simulink model "Appl_DrComfort_CtrlModel"  (R2018b)
settings: configuration reference "CodeConfig_10_ms" (kept outside this file)
undefined symbols (not defined in the file): D_Active, D_CLOSE, D_Inactive, D_InitDelayTime, D_OPEN, D_SoftDistanceDrLegnth, D_WelcomeDistance, FALSE, TRUE
libraries: DareLib x50, simulink x1
(part 1 of 2)
settings Model: Creator=Administrator  LastModifiedBy=Administrator
settings ConfigSetRef: SourceLocation=Base Workspace

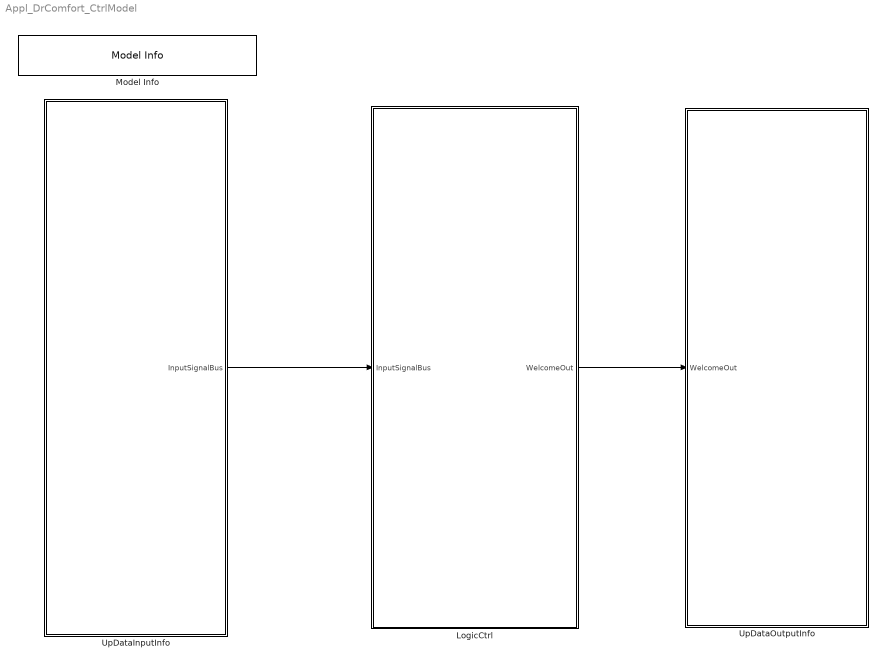
== system Appl_DrComfort_CtrlModel ==
  LogicCtrl : Subsystem  Priority=2  TreatAsAtomicUnit=on
      settings: RTWSystemCode=Nonreusable function  RTWFcnNameOpts=Use subsystem name
  Model Info : simulink/Model-Wide Utilities/Model Info  Frame=on  DisplayStringWithTags=Version：%<ModelVersion>  HorizontalTextAlignment=Center  LeftAlignmentValue=0.5
  UpDataInputInfo : Subsystem  Priority=1  TreatAsAtomicUnit=on
      settings: RTWSystemCode=Nonreusable function  RTWFcnNameOpts=Use subsystem name
  UpDataOutputInfo : Subsystem  Priority=3  TreatAsAtomicUnit=on
      settings: RTWSystemCode=Nonreusable function  RTWFcnNameOpts=Use subsystem name
  wires:
  LogicCtrl/1(WelcomeOut) -> UpDataOutputInfo/1(WelcomeOut)
  UpDataInputInfo/1(InputSignalBus) -> LogicCtrl/1(InputSignalBus)

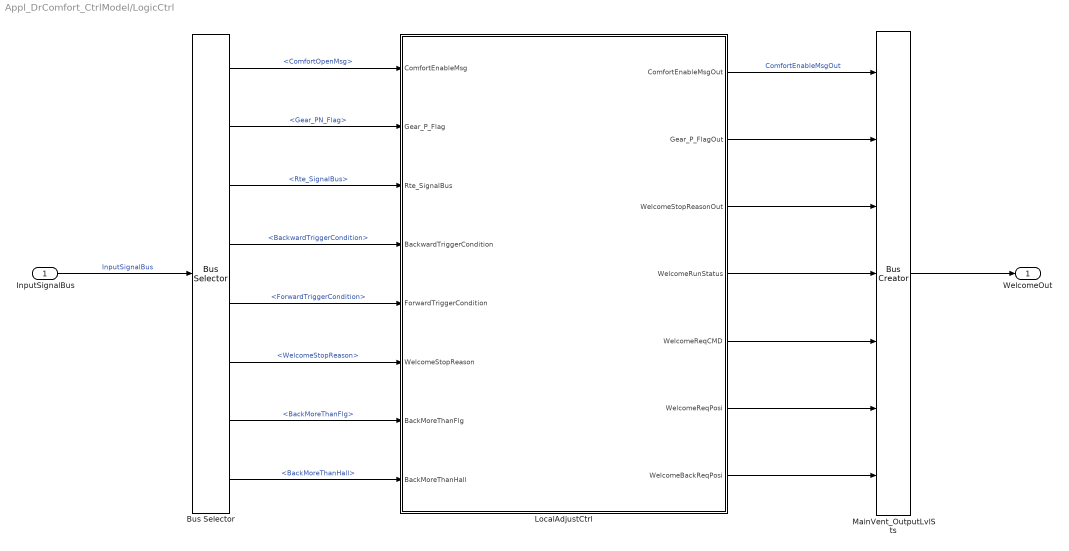
== system Appl_DrComfort_CtrlModel/LogicCtrl ==
  InputSignalBus : Inport
  Bus Selector : BusSelector  OutputSignals=ComfortOpenMsg,Gear_PN_Flag,Rte_SignalBus,BackwardTriggerCondition,ForwardTriggerCondition,WelcomeStopReason,BackMoreThanFlg,BackMoreThanHall
  LocalAdjustCtrl : Subsystem  Description=加热逻辑处理
      settings: AttributesFormatString=%<Description>
  MainVent_OutputLvlSts : BusCreator  Inputs=7
  WelcomeOut : Outport
  wires:
  InputSignalBus/1 -> Bus Selector/1  "InputSignalBus"
  MainVent_OutputLvlSts/1 -> WelcomeOut/1
  Bus Selector/3 -> LocalAdjustCtrl/3(Rte_SignalBus)  "<Rte_SignalBus>"
  Bus Selector/2 -> LocalAdjustCtrl/2(Gear_P_Flag)  "<Gear_PN_Flag>"
  Bus Selector/4 -> LocalAdjustCtrl/4(BackwardTriggerCondition)  "<BackwardTriggerCondition>"
  Bus Selector/5 -> LocalAdjustCtrl/5(ForwardTriggerCondition)  "<ForwardTriggerCondition>"
  Bus Selector/6 -> LocalAdjustCtrl/6(WelcomeStopReason)  "<WelcomeStopReason>"
  LocalAdjustCtrl/2(Gear_P_FlagOut) -> MainVent_OutputLvlSts/2
  LocalAdjustCtrl/3(WelcomeStopReasonOut) -> MainVent_OutputLvlSts/3
  LocalAdjustCtrl/4(WelcomeRunStatus) -> MainVent_OutputLvlSts/4
  LocalAdjustCtrl/5(WelcomeReqCMD) -> MainVent_OutputLvlSts/5
  LocalAdjustCtrl/6(WelcomeReqPosi) -> MainVent_OutputLvlSts/6
  Bus Selector/1 -> LocalAdjustCtrl/1(ComfortEnableMsg)  "<ComfortOpenMsg>"
  LocalAdjustCtrl/1(ComfortEnableMsgOut) -> MainVent_OutputLvlSts/1  "ComfortEnableMsgOut"
  Bus Selector/7 -> LocalAdjustCtrl/7(BackMoreThanFlg)  "<BackMoreThanFlg>"
  Bus Selector/8 -> LocalAdjustCtrl/8(BackMoreThanHall)  "<BackMoreThanHall>"
  LocalAdjustCtrl/7(WelcomeBackReqPosi) -> MainVent_OutputLvlSts/7

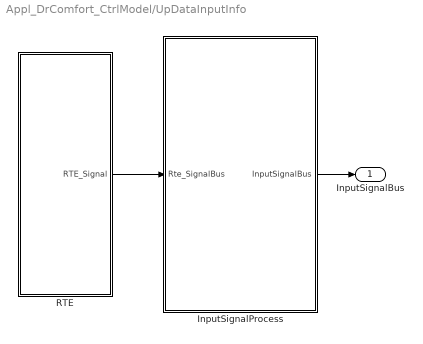
== system Appl_DrComfort_CtrlModel/UpDataInputInfo ==
  InputSignalProcess : Subsystem  Description=数据处理
      settings: AttributesFormatString=%<Description>  RTWSystemCode=Nonreusable function  RTWFcnNameOpts=Use subsystem name
  RTE : Subsystem  Description=接口自动生成  TreatAsAtomicUnit=on
      settings: AttributesFormatString=%<Description>  RTWSystemCode=Nonreusable function  RTWFcnNameOpts=Use subsystem name
  InputSignalBus : Outport
  wires:
  RTE/1(RTE_Signal) -> InputSignalProcess/1(Rte_SignalBus)
  InputSignalProcess/1(InputSignalBus) -> InputSignalBus/1

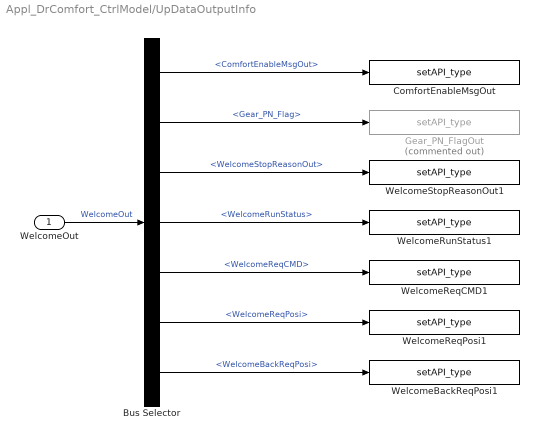
== system Appl_DrComfort_CtrlModel/UpDataOutputInfo ==
  WelcomeOut : Inport
  Bus Selector : BusSelector  OutputSignals=ComfortEnableMsgOut,Gear_PN_Flag,WelcomeStopReasonOut,WelcomeRunStatus,WelcomeReqCMD,WelcomeReqPosi,WelcomeBackReqPosi
  ComfortEnableMsgOut : DareLib/Dare/setAPI_type  g_funcname=CanTx_0x3B2_DSM_St_FLSeatmeet  g_param=""  g_type=uint8  g_size=-1
      settings: AttributesFormatString=%<g_funcname>  SourceProductName=Dare Library
  Gear_PN_FlagOut : DareLib/Dare/setAPI_type  Commented=on  g_funcname=Srvl_Set_D_SimuIndex_GearPN  g_param=D_SimuIndex_GearPN  g_type=uint8  g_size=-1
      settings: AttributesFormatString=%<g_funcname>  SourceProductName=Dare Library
  WelcomeBackReqPosi1 : DareLib/Dare/setAPI_type  g_funcname=Rte_SetVfb_DrWelBackReqPosi  g_param=""  g_type=uint16  g_size=-1
      settings: AttributesFormatString=%<g_funcname>  SourceProductName=Dare Library
  WelcomeReqCMD1 : DareLib/Dare/setAPI_type  g_funcname=Rte_SetVfb_DrWelLengthReqCMD  g_param=""  g_type=uint8  g_size=-1
      settings: AttributesFormatString=%<g_funcname>  SourceProductName=Dare Library
  WelcomeReqPosi1 : DareLib/Dare/setAPI_type  g_funcname=Rte_SetVfb_DrWelLengthReqPosi  g_param=""  g_type=uint16  g_size=-1
      settings: AttributesFormatString=%<g_funcname>  SourceProductName=Dare Library
  WelcomeRunStatus1 : DareLib/Dare/setAPI_type  g_funcname=Rte_SetVfb_DrWelcomeRunSts  g_param=""  g_type=uint8  g_size=-1
      settings: AttributesFormatString=%<g_funcname>  SourceProductName=Dare Library
  WelcomeStopReasonOut1 : DareLib/Dare/setAPI_type  g_funcname=Rte_SetVfb_DrWelcomeStopReason  g_param=""  g_type=uint8  g_size=-1
      settings: AttributesFormatString=%<g_funcname>  SourceProductName=Dare Library
  wires:
  WelcomeOut/1 -> Bus Selector/1  "WelcomeOut"
  Bus Selector/5 -> WelcomeReqCMD1/1  "<WelcomeReqCMD>"
  Bus Selector/4 -> WelcomeRunStatus1/1  "<WelcomeRunStatus>"
  Bus Selector/3 -> WelcomeStopReasonOut1/1  "<WelcomeStopReasonOut>"
  Bus Selector/2 -> Gear_PN_FlagOut/1  "<Gear_PN_Flag>"
  Bus Selector/6 -> WelcomeReqPosi1/1  "<WelcomeReqPosi>"
  Bus Selector/1 -> ComfortEnableMsgOut/1  "<ComfortEnableMsgOut>"
  Bus Selector/7 -> WelcomeBackReqPosi1/1  "<WelcomeBackReqPosi>"

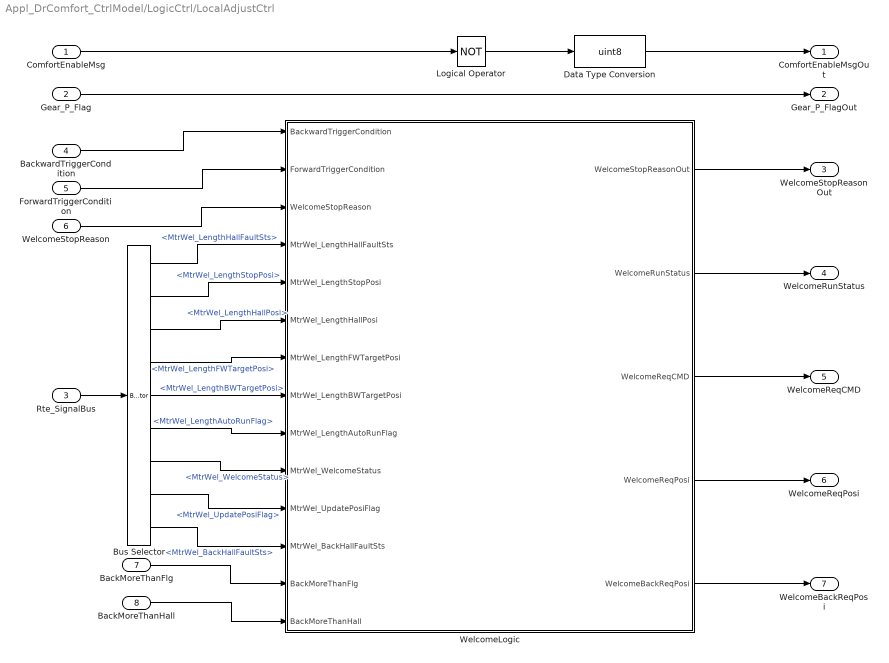
== system Appl_DrComfort_CtrlModel/LogicCtrl/LocalAdjustCtrl ==
  ComfortEnableMsg : Inport
  Gear_P_Flag : Inport  Port=2
  Rte_SignalBus : Inport  Port=3
  BackwardTriggerCondition : Inport  Port=4
  ForwardTriggerCondition : Inport  Port=5
  WelcomeStopReason : Inport  Port=6
  BackMoreThanFlg : Inport  Port=7
  BackMoreThanHall : Inport  Port=8
  Bus Selector : BusSelector  OutputSignals=MtrWel_LengthHallFaultSts,MtrWel_LengthStopPosi,MtrWel_LengthHallPosi,MtrWel_LengthFWTargetPosi,MtrWel_LengthBWTargetPosi,MtrWel_LengthAutoRunFlag,MtrWel_WelcomeStatus,MtrWel_UpdatePosiFlag,MtrWel_BackHallFaultSts
  Data Type Conversion : DataTypeConversion  OutDataTypeStr=uint8
  Logical Operator : Logic  Operator=NOT  AllPortsSameDT=off  OutDataTypeStr=boolean
  WelcomeLogic : Stateflow chart  TreatAsAtomicUnit=on
  ComfortEnableMsgOut : Outport
  Gear_P_FlagOut : Outport  Port=2
  WelcomeStopReasonOut : Outport  Port=3
  WelcomeRunStatus : Outport  Port=4
  WelcomeReqCMD : Outport  Port=5
  WelcomeReqPosi : Outport  Port=6
  WelcomeBackReqPosi : Outport  Port=7
  wires:
  Gear_P_Flag/1 -> Gear_P_FlagOut/1
  Rte_SignalBus/1 -> Bus Selector/1
  BackwardTriggerCondition/1 -> WelcomeLogic/1(BackwardTriggerCondition)
  ForwardTriggerCondition/1 -> WelcomeLogic/2(ForwardTriggerCondition)
  WelcomeStopReason/1 -> WelcomeLogic/3(WelcomeStopReason)
  Bus Selector/2 -> WelcomeLogic/5(MtrWel_LengthStopPosi)  "<MtrWel_LengthStopPosi>"
  Bus Selector/3 -> WelcomeLogic/6(MtrWel_LengthHallPosi)  "<MtrWel_LengthHallPosi>"
  Bus Selector/6 -> WelcomeLogic/9(MtrWel_LengthAutoRunFlag)  "<MtrWel_LengthAutoRunFlag>"
  Bus Selector/4 -> WelcomeLogic/7(MtrWel_LengthFWTargetPosi)  "<MtrWel_LengthFWTargetPosi>"
  Bus Selector/5 -> WelcomeLogic/8(MtrWel_LengthBWTargetPosi)  "<MtrWel_LengthBWTargetPosi>"
  Bus Selector/7 -> WelcomeLogic/10(MtrWel_WelcomeStatus)  "<MtrWel_WelcomeStatus>"
  WelcomeLogic/1(WelcomeStopReasonOut) -> WelcomeStopReasonOut/1
  WelcomeLogic/2(WelcomeRunStatus) -> WelcomeRunStatus/1
  WelcomeLogic/3(WelcomeReqCMD) -> WelcomeReqCMD/1
  WelcomeLogic/4(WelcomeReqPosi) -> WelcomeReqPosi/1
  Logical Operator/1 -> Data Type Conversion/1
  ComfortEnableMsg/1 -> Logical Operator/1
  Data Type Conversion/1 -> ComfortEnableMsgOut/1
  Bus Selector/1 -> WelcomeLogic/4(MtrWel_LengthHallFaultSts)  "<MtrWel_LengthHallFaultSts>"
  Bus Selector/8 -> WelcomeLogic/11(MtrWel_UpdatePosiFlag)  "<MtrWel_UpdatePosiFlag>"
  BackMoreThanHall/1 -> WelcomeLogic/14(BackMoreThanHall)
  BackMoreThanFlg/1 -> WelcomeLogic/13(BackMoreThanFlg)
  Bus Selector/9 -> WelcomeLogic/12(MtrWel_BackHallFaultSts)  "<MtrWel_BackHallFaultSts>"
  WelcomeLogic/5(WelcomeBackReqPosi) -> WelcomeBackReqPosi/1

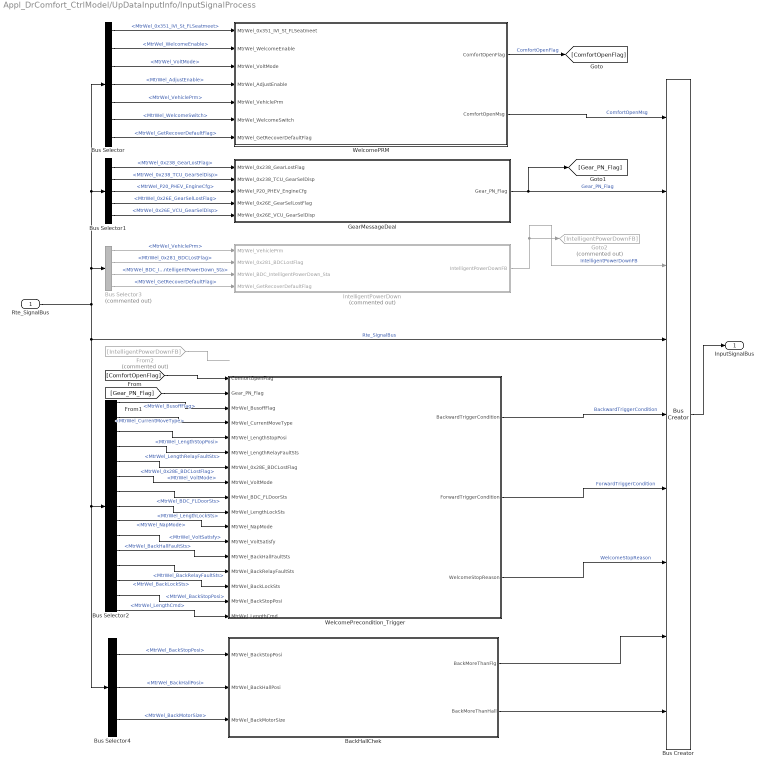
== system Appl_DrComfort_CtrlModel/UpDataInputInfo/InputSignalProcess ==
  Rte_SignalBus : Inport
  "BackHallChek " : Subsystem
  Bus Creator : BusCreator  Inputs=9
  Bus Selector : BusSelector  OutputSignals=MtrWel_0x351_IVI_St_FLSeatmeet,MtrWel_WelcomeEnable,MtrWel_VoltMode,MtrWel_AdjustEnable,MtrWel_VehiclePrm,MtrWel_WelcomeSwitch,MtrWel_GetRecoverDefaultFlag
  Bus Selector1 : BusSelector  OutputSignals=MtrWel_0x238_GearLostFlag,MtrWel_0x238_TCU_GearSelDisp,MtrWel_P20_PHEV_EngineCfg,MtrWel_0x26E_GearSelLostFlag,MtrWel_0x26E_VCU_GearSelDisp
  Bus Selector2 : BusSelector  OutputSignals=MtrWel_BusoffFlag,MtrWel_CurrentMoveType,MtrWel_LengthStopPosi,MtrWel_LengthRelayFaultSts,MtrWel_0x28E_BDCLostFlag,MtrWel_VoltMode,MtrWel_BDC_FLDoorSts,MtrWel_LengthLockSts,MtrWel_NapMode,MtrWel_VoltSatisfy,MtrWel_BackHallFaultSts,MtrWel_BackRelayFaultSts,MtrWel_BackLockSts,MtrWel_BackStopPosi,MtrWel_LengthCmd
  Bus Selector3 : BusSelector  Commented=on  OutputSignals=MtrWel_VehiclePrm,MtrWel_0x281_BDCLostFlag,MtrWel_BDC_IntelligentPowerDown_Sta,MtrWel_GetRecoverDefaultFlag
  Bus Selector4 : BusSelector  OutputSignals=MtrWel_BackStopPosi,MtrWel_BackHallPosi,MtrWel_BackMotorSize
  From2 : From  Commented=on  GotoTag=IntelligentPowerDownFB
  GearMessageDeal : Subsystem  Description=档位报文处理
      settings: AttributesFormatString=%<Description>
  Goto2 : Goto  Commented=on  GotoTag=IntelligentPowerDownFB
  IntelligentPowerDown : Subsystem  Description=智能下电处理  Commented=on
      settings: AttributesFormatString=%<Description>
  WelcomePRM : Subsystem  Description=迎宾配置
      settings: AttributesFormatString=%<Description>
  WelcomePrecondition_Trigger : Subsystem  Description=迎宾前置条件_触发条件
      settings: AttributesFormatString=%<Description>
  InputSignalBus : Outport
  wires:
  Bus Creator/1 -> InputSignalBus/1
  Rte_SignalBus/1 -> Bus Selector4/1, Bus Selector2/1, Bus Creator/4, Bus Selector/1, Bus Selector1/1, Bus Selector3/1  "Rte_SignalBus"
  WelcomePRM/1(ComfortOpenFlag) -> [ComfortOpenFlag]  "ComfortOpenFlag"
  Bus Selector/1 -> WelcomePRM/1(MtrWel_0x351_IVI_St_FLSeatmeet)  "<MtrWel_0x351_IVI_St_FLSeatmeet>"
  Bus Selector/2 -> WelcomePRM/2(MtrWel_WelcomeEnable)  "<MtrWel_WelcomeEnable>"
  Bus Selector/3 -> WelcomePRM/3(MtrWel_VoltMode)  "<MtrWel_VoltMode>"
  Bus Selector1/1 -> GearMessageDeal/1(MtrWel_0x238_GearLostFlag)  "<MtrWel_0x238_GearLostFlag>"
  Bus Selector1/2 -> GearMessageDeal/2(MtrWel_0x238_TCU_GearSelDisp)  "<MtrWel_0x238_TCU_GearSelDisp>"
  GearMessageDeal/1(Gear_PN_Flag) -> [Gear_PN_Flag], Bus Creator/2  "Gear_PN_Flag"
  Bus Selector2/1 -> WelcomePrecondition_Trigger/3(MtrWel_BusoffFlag)  "<MtrWel_BusoffFlag>"
  [Gear_PN_Flag] -> WelcomePrecondition_Trigger/2(Gear_PN_Flag)
  [ComfortOpenFlag] -> WelcomePrecondition_Trigger/1(ComfortOpenFlag)
  WelcomePrecondition_Trigger/1(BackwardTriggerCondition) -> Bus Creator/5  "BackwardTriggerCondition"
  WelcomePrecondition_Trigger/2(ForwardTriggerCondition) -> Bus Creator/6  "ForwardTriggerCondition"
  WelcomePrecondition_Trigger/3(WelcomeStopReason) -> Bus Creator/7  "WelcomeStopReason"
  Bus Selector2/2 -> WelcomePrecondition_Trigger/4(MtrWel_CurrentMoveType)  "<MtrWel_CurrentMoveType>"
  Bus Selector/4 -> WelcomePRM/4(MtrWel_AdjustEnable)  "<MtrWel_AdjustEnable>"
  Bus Selector/5 -> WelcomePRM/5(MtrWel_VehiclePrm)  "<MtrWel_VehiclePrm>"
  Bus Selector/6 -> WelcomePRM/6(MtrWel_WelcomeSwitch)  "<MtrWel_WelcomeSwitch>"
  Bus Selector/7 -> WelcomePRM/7(MtrWel_GetRecoverDefaultFlag)  "<MtrWel_GetRecoverDefaultFlag>"
  Bus Selector3/2 -> IntelligentPowerDown/2(MtrWel_0x281_BDCLostFlag)  "<MtrWel_0x281_BDCLostFlag>"
  Bus Selector3/3 -> IntelligentPowerDown/3(MtrWel_BDC_IntelligentPowerDown_Sta)  "<MtrWel_BDC_IntelligentPowerDown_Sta>"
  Bus Selector3/1 -> IntelligentPowerDown/1(MtrWel_VehiclePrm)  "<MtrWel_VehiclePrm>"
  IntelligentPowerDown/1(IntelligentPowerDownFB) -> Goto2/1, Bus Creator/3  "IntelligentPowerDownFB"
  From2/1 -> ?
  Bus Selector2/3 -> WelcomePrecondition_Trigger/5(MtrWel_LengthStopPosi)  "<MtrWel_LengthStopPosi>"
  Bus Selector2/4 -> WelcomePrecondition_Trigger/6(MtrWel_LengthRelayFaultSts)  "<MtrWel_LengthRelayFaultSts>"
  Bus Selector3/4 -> IntelligentPowerDown/4(MtrWel_GetRecoverDefaultFlag)  "<MtrWel_GetRecoverDefaultFlag>"
  Bus Selector2/5 -> WelcomePrecondition_Trigger/7(MtrWel_0x28E_BDCLostFlag)  "<MtrWel_0x28E_BDCLostFlag>"
  Bus Selector2/6 -> WelcomePrecondition_Trigger/8(MtrWel_VoltMode)  "<MtrWel_VoltMode>"
  Bus Selector2/7 -> WelcomePrecondition_Trigger/9(MtrWel_BDC_FLDoorSts)  "<MtrWel_BDC_FLDoorSts>"
  WelcomePRM/2(ComfortOpenMsg) -> Bus Creator/1  "ComfortOpenMsg"
  Bus Selector2/8 -> WelcomePrecondition_Trigger/10(MtrWel_LengthLockSts)  "<MtrWel_LengthLockSts>"
  Bus Selector2/9 -> WelcomePrecondition_Trigger/11(MtrWel_NapMode)  "<MtrWel_NapMode>"
  Bus Selector1/3 -> GearMessageDeal/3(MtrWel_P20_PHEV_EngineCfg)  "<MtrWel_P20_PHEV_EngineCfg>"
  Bus Selector1/4 -> GearMessageDeal/4(MtrWel_0x26E_GearSelLostFlag)  "<MtrWel_0x26E_GearSelLostFlag>"
  Bus Selector1/5 -> GearMessageDeal/5(MtrWel_0x26E_VCU_GearSelDisp)  "<MtrWel_0x26E_VCU_GearSelDisp>"
  Bus Selector2/10 -> WelcomePrecondition_Trigger/12(MtrWel_VoltSatisfy)  "<MtrWel_VoltSatisfy>"
  Bus Selector2/11 -> WelcomePrecondition_Trigger/13(MtrWel_BackHallFaultSts)  "<MtrWel_BackHallFaultSts>"
  Bus Selector2/12 -> WelcomePrecondition_Trigger/14(MtrWel_BackRelayFaultSts)  "<MtrWel_BackRelayFaultSts>"
  Bus Selector2/13 -> WelcomePrecondition_Trigger/15(MtrWel_BackLockSts)  "<MtrWel_BackLockSts>"
  Bus Selector2/14 -> WelcomePrecondition_Trigger/16(MtrWel_BackStopPosi)  "<MtrWel_BackStopPosi>"
  "BackHallChek "/1(BackMoreThanFlg) -> Bus Creator/8
  "BackHallChek "/2(BackMoreThanHall) -> Bus Creator/9
  Bus Selector4/1 -> "BackHallChek "/1(MtrWel_BackStopPosi)  "<MtrWel_BackStopPosi>"
  Bus Selector4/2 -> "BackHallChek "/2(MtrWel_BackHallPosi)  "<MtrWel_BackHallPosi>"
  Bus Selector4/3 -> "BackHallChek "/3(MtrWel_BackMotorSize)  "<MtrWel_BackMotorSize>"
  Bus Selector2/15 -> WelcomePrecondition_Trigger/17(MtrWel_LengthCmd)  "<MtrWel_LengthCmd>"

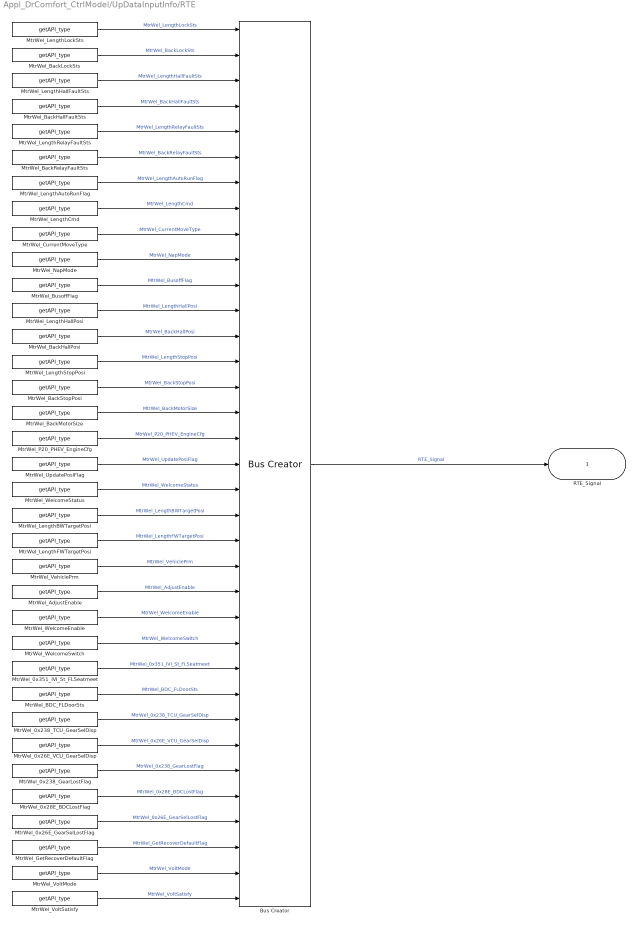
== system Appl_DrComfort_CtrlModel/UpDataInputInfo/RTE ==
  Bus Creator : BusCreator  Inputs=35
  MtrWel_0x238_GearLostFlag : DareLib/Dare/getAPI_type  g_funcname=Ecual_GetCanMsgLostFlag  g_param=eRXINDEX_0x238  g_type=uint8  g_size=-1
      settings: AttributesFormatString=%<g_funcname>  SourceProductName=Dare Library
  MtrWel_0x238_TCU_GearSelDisp : DareLib/Dare/getAPI_type  g_funcname=CanRx_0x238_TCU_GearSelDisp  g_param=""  g_type=uint8  g_size=-1
      settings: AttributesFormatString=%<g_funcname>  SourceProductName=Dare Library
  MtrWel_0x26E_GearSelLostFlag : DareLib/Dare/getAPI_type  g_funcname=Ecual_GetCanMsgLostFlag  g_param=eRXINDEX_0x26E  g_type=uint8  g_size=-1
      settings: AttributesFormatString=%<g_funcname>  SourceProductName=Dare Library
  MtrWel_0x26E_VCU_GearSelDisp : DareLib/Dare/getAPI_type  g_funcname=CanRx_0x26E_VCU_GearSelDisp  g_param=""  g_type=uint8  g_size=-1
      settings: AttributesFormatString=%<g_funcname>  SourceProductName=Dare Library
  MtrWel_0x28E_BDCLostFlag : DareLib/Dare/getAPI_type  g_funcname=Ecual_GetCanMsgLostFlag  g_param=eRXINDEX_0x28E  g_type=uint8  g_size=-1
      settings: AttributesFormatString=%<g_funcname>  SourceProductName=Dare Library
  MtrWel_0x351_IVI_St_FLSeatmeet : DareLib/Dare/getAPI_type  g_funcname=CanRx_0x351_IVI_St_FLSeatmeet  g_param=""  g_type=uint8  g_size=-1
      settings: AttributesFormatString=%<g_funcname>  SourceProductName=Dare Library
  MtrWel_AdjustEnable : DareLib/Dare/getAPI_type  g_funcname=Srvl_GetMemIndexDataU8  g_param=EN_MemIndex_DrAdjustConfig  g_type=uint8  g_enum=enDrAdjustEnable  g_size=-1
      settings: AttributesFormatString=%<g_funcname>  SourceProductName=Dare Library
  MtrWel_BDC_FLDoorSts : DareLib/Dare/getAPI_type  g_funcname=CanRx_0x28E_BDC_FLDoorSts  g_param=""  g_type=uint8  g_size=-1
      settings: AttributesFormatString=%<g_funcname>  SourceProductName=Dare Library
  MtrWel_BackHallFaultSts : DareLib/Dare/getAPI_type  g_funcname=Rte_GetVfb_DrBackHallErr  g_param=""  g_type=uint8  g_size=-1
      settings: AttributesFormatString=%<g_funcname>  SourceProductName=Dare Library
  MtrWel_BackHallPosi : DareLib/Dare/getAPI_type  g_funcname=Cdd_GetCurrentHallCnt  g_param=EN_DriverBack  g_type=uint16  g_size=-1
      settings: AttributesFormatString=%<g_funcname>  SourceProductName=Dare Library
  MtrWel_BackLockSts : DareLib/Dare/getAPI_type  g_funcname=Rte_GetVfb_DrBackStallErr  g_param=""  g_type=uint8  g_size=-1
      settings: AttributesFormatString=%<g_funcname>  SourceProductName=Dare Library
  MtrWel_BackMotorSize : DareLib/Dare/getAPI_type  g_funcname=Cdd_GetMotorSize  g_param=EN_DriverBack  g_type=uint16  g_size=-1
      settings: AttributesFormatString=%<g_funcname>  SourceProductName=Dare Library
  MtrWel_BackRelayFaultSts : DareLib/Dare/getAPI_type  g_funcname=Rte_GetVfb_DrBackRelayAdheErr  g_param=""  g_type=uint8  g_size=-1
      settings: AttributesFormatString=%<g_funcname>  SourceProductName=Dare Library
  MtrWel_BackStopPosi : DareLib/Dare/getAPI_type  g_funcname=Cdd_GetMotorHardStop  g_param=EN_DriverBack  g_type=uint16  g_size=-1
      settings: AttributesFormatString=%<g_funcname>  SourceProductName=Dare Library
  MtrWel_BusoffFlag : DareLib/Dare/getAPI_type  g_funcname=Nm_IsBusOff  g_param=""  g_type=uint8  g_size=-1
      settings: AttributesFormatString=%<g_funcname>  SourceProductName=Dare Library
  MtrWel_CurrentMoveType : DareLib/Dare/getAPI_type  g_funcname=Rte_GetVfb_DrMoveType  g_param=""  g_type=uint8  g_enum=enSeatMotorRunType  g_size=-1
      settings: AttributesFormatString=%<g_funcname>  SourceProductName=Dare Library
  MtrWel_GetRecoverDefaultFlag : DareLib/Dare/getAPI_type  g_funcname=GetRecoverDefaultFlag  g_param=""  g_type=uint8  g_size=-1
      settings: AttributesFormatString=%<g_funcname>  SourceProductName=Dare Library
  MtrWel_LengthAutoRunFlag : DareLib/Dare/getAPI_type  g_funcname=Rte_GetVfb_DrLengthAutoRunFlag  g_param=""  g_type=uint8  g_enum=enSeatAutoRunSts  g_size=-1
      settings: AttributesFormatString=%<g_funcname>  SourceProductName=Dare Library
  MtrWel_LengthBWTargetPosi : DareLib/Dare/getAPI_type  g_funcname=Srvl_GetMemIndexDataU16  g_param=EN_MemIndex_DrWelcome_LenTar_BackWard  g_type=uint16  g_size=-1
      settings: AttributesFormatString=%<g_funcname>  SourceProductName=Dare Library
  MtrWel_LengthCmd : DareLib/Dare/getAPI_type  g_funcname=Rte_GetVfb_DrHeightMotorCmd  g_param=""  g_type=uint8  g_size=-1
      settings: AttributesFormatString=%<g_funcname>  SourceProductName=Dare Library
  MtrWel_LengthFWTargetPosi : DareLib/Dare/getAPI_type  g_funcname=Srvl_GetMemIndexDataU16  g_param=EN_MemIndex_DrWelcome_LenTar_ForWard  g_type=uint16  g_size=-1
      settings: AttributesFormatString=%<g_funcname>  SourceProductName=Dare Library
  MtrWel_LengthHallFaultSts : DareLib/Dare/getAPI_type  g_funcname=Rte_GetVfb_DrLengthHallErr  g_param=""  g_type=uint8  g_size=-1
      settings: AttributesFormatString=%<g_funcname>  SourceProductName=Dare Library
  MtrWel_LengthHallPosi : DareLib/Dare/getAPI_type  g_funcname=Cdd_GetCurrentHallCnt  g_param=EN_DriverLength  g_type=uint16  g_size=-1
      settings: AttributesFormatString=%<g_funcname>  SourceProductName=Dare Library
  MtrWel_LengthLockSts : DareLib/Dare/getAPI_type  g_funcname=Rte_GetVfb_DrLengthStallErr  g_param=""  g_type=uint8  g_size=-1
      settings: AttributesFormatString=%<g_funcname>  SourceProductName=Dare Library
  MtrWel_LengthRelayFaultSts : DareLib/Dare/getAPI_type  g_funcname=Rte_GetVfb_DrLengthRelayAdheErr  g_param=""  g_type=uint8  g_size=-1
      settings: AttributesFormatString=%<g_funcname>  SourceProductName=Dare Library
  MtrWel_LengthStopPosi : DareLib/Dare/getAPI_type  g_funcname=Cdd_GetMotorHardStop  g_param=EN_DriverLength  g_type=uint16  g_size=-1
      settings: AttributesFormatString=%<g_funcname>  SourceProductName=Dare Library
  MtrWel_NapMode : DareLib/Dare/getAPI_type  g_funcname=Rte_GetVfb_NapMode  g_param=""  g_type=uint8  g_enum=enNapMode  g_size=-1
      settings: AttributesFormatString=%<g_funcname>  SourceProductName=Dare Library
  MtrWel_P20_PHEV_EngineCfg : DareLib/Dare/getAPI_type  g_funcname=Srvl_GetMemIndexDataU8  g_param=EN_MemIndex_Heat_P20_PHEV_EngineCfg  g_type=uint8  g_size=-1
      settings: AttributesFormatString=%<g_funcname>  SourceProductName=Dare Library
  MtrWel_UpdatePosiFlag : DareLib/Dare/getAPI_type  g_funcname=Srvl_GetMemIndexDataU8  g_param=EN_MemIndex_WelcomeDrUpate  g_type=uint8  g_size=-1
      settings: AttributesFormatString=%<g_funcname>  SourceProductName=Dare Library
  MtrWel_VehiclePrm : DareLib/Dare/getAPI_type  g_funcname=Srvl_GetMemIndexDataU8  g_param=EN_MemIndex_Heat_CarType  g_type=uint8  g_enum=enVehTypePrm  g_size=-1
      settings: AttributesFormatString=%<g_funcname>  SourceProductName=Dare Library
  MtrWel_VoltMode : DareLib/Dare/getAPI_type  g_funcname=Rte_GetVfb_VoltMode  g_param=""  g_type=uint8  g_enum=enFinalPowerMode  g_size=-1
      settings: AttributesFormatString=%<g_funcname>  SourceProductName=Dare Library
  MtrWel_VoltSatisfy : DareLib/Dare/getAPI_type  g_funcname=Rte_GetVfb_VoltSatisfy  g_param=""  g_type=uint8  g_size=-1
      settings: AttributesFormatString=%<g_funcname>  SourceProductName=Dare Library
  MtrWel_WelcomeEnable : DareLib/Dare/getAPI_type  g_funcname=Srvl_GetMemIndexDataU8  g_param=EN_MemIndex_DrMemoryConfig  g_type=uint8  g_size=-1
      settings: AttributesFormatString=%<g_funcname>  SourceProductName=Dare Library
  MtrWel_WelcomeStatus : DareLib/Dare/getAPI_type  g_funcname=Srvl_GetMemIndexDataU8  g_param=EN_MemIndex_WelcomeStatus  g_type=uint8  g_enum=enWelcomeSts  g_size=-1
      settings: AttributesFormatString=%<g_funcname>  SourceProductName=Dare Library
  MtrWel_WelcomeSwitch : DareLib/Dare/getAPI_type  g_funcname=Srvl_GetMemIndexDataU8  g_param=EN_MemIndex_WelcomeSwitch  g_type=uint8  g_size=-1
      settings: AttributesFormatString=%<g_funcname>  SourceProductName=Dare Library
  RTE_Signal : Outport
  wires:
  Bus Creator/1 -> RTE_Signal/1  "RTE_Signal"
  MtrWel_LengthLockSts/1 -> Bus Creator/1  "MtrWel_LengthLockSts"
  MtrWel_BackLockSts/1 -> Bus Creator/2  "MtrWel_BackLockSts"
  MtrWel_LengthHallFaultSts/1 -> Bus Creator/3  "MtrWel_LengthHallFaultSts"
  MtrWel_BackHallFaultSts/1 -> Bus Creator/4  "MtrWel_BackHallFaultSts"
  MtrWel_LengthRelayFaultSts/1 -> Bus Creator/5  "MtrWel_LengthRelayFaultSts"
  MtrWel_BackRelayFaultSts/1 -> Bus Creator/6  "MtrWel_BackRelayFaultSts"
  MtrWel_LengthAutoRunFlag/1 -> Bus Creator/7  "MtrWel_LengthAutoRunFlag"
  MtrWel_LengthCmd/1 -> Bus Creator/8  "MtrWel_LengthCmd"
  MtrWel_CurrentMoveType/1 -> Bus Creator/9  "MtrWel_CurrentMoveType"
  MtrWel_NapMode/1 -> Bus Creator/10  "MtrWel_NapMode"
  MtrWel_BusoffFlag/1 -> Bus Creator/11  "MtrWel_BusoffFlag"
  MtrWel_LengthHallPosi/1 -> Bus Creator/12  "MtrWel_LengthHallPosi"
  MtrWel_BackHallPosi/1 -> Bus Creator/13  "MtrWel_BackHallPosi"
  MtrWel_LengthStopPosi/1 -> Bus Creator/14  "MtrWel_LengthStopPosi"
  MtrWel_BackStopPosi/1 -> Bus Creator/15  "MtrWel_BackStopPosi"
  MtrWel_BackMotorSize/1 -> Bus Creator/16  "MtrWel_BackMotorSize"
  MtrWel_P20_PHEV_EngineCfg/1 -> Bus Creator/17  "MtrWel_P20_PHEV_EngineCfg"
  MtrWel_UpdatePosiFlag/1 -> Bus Creator/18  "MtrWel_UpdatePosiFlag"
  MtrWel_WelcomeStatus/1 -> Bus Creator/19  "MtrWel_WelcomeStatus"
  MtrWel_LengthBWTargetPosi/1 -> Bus Creator/20  "MtrWel_LengthBWTargetPosi"
  MtrWel_LengthFWTargetPosi/1 -> Bus Creator/21  "MtrWel_LengthFWTargetPosi"
  MtrWel_VehiclePrm/1 -> Bus Creator/22  "MtrWel_VehiclePrm"
  MtrWel_AdjustEnable/1 -> Bus Creator/23  "MtrWel_AdjustEnable"
  MtrWel_WelcomeEnable/1 -> Bus Creator/24  "MtrWel_WelcomeEnable"
  MtrWel_WelcomeSwitch/1 -> Bus Creator/25  "MtrWel_WelcomeSwitch"
  MtrWel_0x351_IVI_St_FLSeatmeet/1 -> Bus Creator/26  "MtrWel_0x351_IVI_St_FLSeatmeet"
  MtrWel_BDC_FLDoorSts/1 -> Bus Creator/27  "MtrWel_BDC_FLDoorSts"
  MtrWel_0x238_TCU_GearSelDisp/1 -> Bus Creator/28  "MtrWel_0x238_TCU_GearSelDisp"
  MtrWel_0x26E_VCU_GearSelDisp/1 -> Bus Creator/29  "MtrWel_0x26E_VCU_GearSelDisp"
  MtrWel_0x238_GearLostFlag/1 -> Bus Creator/30  "MtrWel_0x238_GearLostFlag"
  MtrWel_0x28E_BDCLostFlag/1 -> Bus Creator/31  "MtrWel_0x28E_BDCLostFlag"
  MtrWel_0x26E_GearSelLostFlag/1 -> Bus Creator/32  "MtrWel_0x26E_GearSelLostFlag"
  MtrWel_GetRecoverDefaultFlag/1 -> Bus Creator/33  "MtrWel_GetRecoverDefaultFlag"
  MtrWel_VoltMode/1 -> Bus Creator/34  "MtrWel_VoltMode"
  MtrWel_VoltSatisfy/1 -> Bus Creator/35  "MtrWel_VoltSatisfy"

== system Appl_DrComfort_CtrlModel/LogicCtrl/LocalAdjustCtrl/WelcomeLogic/Set_WelcomeBWTargertPosi ==
  In1 : Inport
  f : TriggerPort  TriggerType=function-call  VariantControl=(inherit)
      settings: CopyFcn=Stateflow.SLINSF.SimulinkMan.removeBlockPreDeleteFcn  PreDeleteFcn=Stateflow.SLINSF.SimulinkMan.unsafePredeleteFcn
  setAPI_type : DareLib/Dare/setAPI_type  g_funcname=Srvl_SetMemIndexDataU16  g_param=EN_MemIndex_DrWelcome_LenTar_BackWard  g_type=uint16  g_size=-1
      settings: AttributesFormatString=%<g_funcname>  SourceProductName=Dare Library
  wires:
  In1/1 -> setAPI_type/1

== system Appl_DrComfort_CtrlModel/LogicCtrl/LocalAdjustCtrl/WelcomeLogic/Set_WelcomeFWTargertPosi ==
  In1 : Inport
  f : TriggerPort  TriggerType=function-call  VariantControl=(inherit)
      settings: CopyFcn=Stateflow.SLINSF.SimulinkMan.removeBlockPreDeleteFcn  PreDeleteFcn=Stateflow.SLINSF.SimulinkMan.unsafePredeleteFcn
  setAPI_type : DareLib/Dare/setAPI_type  g_funcname=Srvl_SetMemIndexDataU16  g_param=EN_MemIndex_DrWelcome_LenTar_ForWard  g_type=uint16  g_size=-1
      settings: AttributesFormatString=%<g_funcname>  SourceProductName=Dare Library
  wires:
  In1/1 -> setAPI_type/1

== system Appl_DrComfort_CtrlModel/LogicCtrl/LocalAdjustCtrl/WelcomeLogic/Set_WelcomeStatus ==
  In1 : Inport
  f : TriggerPort  TriggerType=function-call  VariantControl=(inherit)
      settings: CopyFcn=Stateflow.SLINSF.SimulinkMan.removeBlockPreDeleteFcn  PreDeleteFcn=Stateflow.SLINSF.SimulinkMan.unsafePredeleteFcn
  setAPI_type : DareLib/Dare/setAPI_type  g_funcname=Srvl_SetMemIndexDataU8  g_param=EN_MemIndex_WelcomeStatus  g_type=uint8  g_size=-1
      settings: AttributesFormatString=%<g_funcname>  SourceProductName=Dare Library
  wires:
  In1/1 -> setAPI_type/1

== system Appl_DrComfort_CtrlModel/LogicCtrl/LocalAdjustCtrl/WelcomeLogic/Set_WelcomeUpdatePosiFlag ==
  In1 : Inport
  f : TriggerPort  TriggerType=function-call  VariantControl=(inherit)
      settings: CopyFcn=Stateflow.SLINSF.SimulinkMan.removeBlockPreDeleteFcn  PreDeleteFcn=Stateflow.SLINSF.SimulinkMan.unsafePredeleteFcn
  setAPI_type : DareLib/Dare/setAPI_type  g_funcname=Srvl_SetMemIndexDataU8  g_param=EN_MemIndex_WelcomeDrUpate  g_type=uint16  g_size=-1
      settings: AttributesFormatString=%<g_funcname>  SourceProductName=Dare Library
  wires:
  In1/1 -> setAPI_type/1

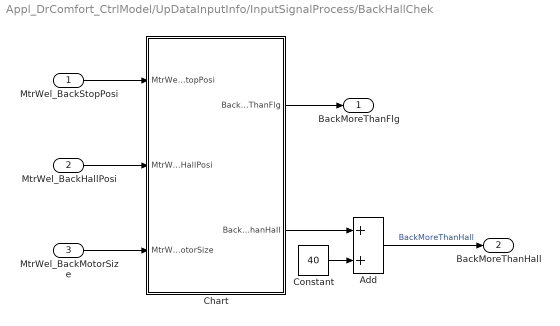
== system Appl_DrComfort_CtrlModel/UpDataInputInfo/InputSignalProcess/BackHallChek  ==
  MtrWel_BackStopPosi : Inport
  MtrWel_BackHallPosi : Inport  Port=2
  MtrWel_BackMotorSize : Inport  Port=3
  Add : Sum  AccumDataTypeStr=uint16
  Chart : Stateflow chart  TreatAsAtomicUnit=on
  Constant : Constant  Value=40  OutDataTypeStr=uint16
  BackMoreThanFlg : Outport
  BackMoreThanHall : Outport  Port=2
  wires:
  MtrWel_BackStopPosi/1 -> Chart/1(MtrWel_BackStopPosi)
  MtrWel_BackHallPosi/1 -> Chart/2(MtrWel_BackHallPosi)
  MtrWel_BackMotorSize/1 -> Chart/3(MtrWel_BackMotorSize)
  Chart/1(BackMoreThanFlg) -> BackMoreThanFlg/1
  Chart/2(BackMoreThanHall) -> Add/1
  Constant/1 -> Add/2
  Add/1 -> BackMoreThanHall/1  "BackMoreThanHall"

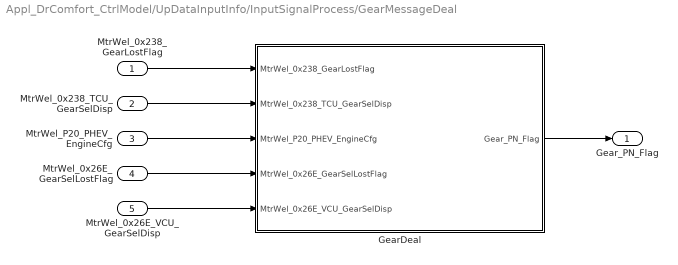
== system Appl_DrComfort_CtrlModel/UpDataInputInfo/InputSignalProcess/GearMessageDeal ==
  MtrWel_0x238_GearLostFlag : Inport
  MtrWel_0x238_TCU_GearSelDisp : Inport  Port=2
  MtrWel_P20_PHEV_EngineCfg : Inport  Port=3
  MtrWel_0x26E_GearSelLostFlag : Inport  Port=4
  MtrWel_0x26E_VCU_GearSelDisp : Inport  Port=5
  GearDeal : Stateflow chart  TreatAsAtomicUnit=on
  Gear_PN_Flag : Outport
  wires:
  MtrWel_0x238_GearLostFlag/1 -> GearDeal/1(MtrWel_0x238_GearLostFlag)
  MtrWel_0x238_TCU_GearSelDisp/1 -> GearDeal/2(MtrWel_0x238_TCU_GearSelDisp)
  GearDeal/1(Gear_PN_Flag) -> Gear_PN_Flag/1
  MtrWel_P20_PHEV_EngineCfg/1 -> GearDeal/3(MtrWel_P20_PHEV_EngineCfg)
  MtrWel_0x26E_GearSelLostFlag/1 -> GearDeal/4(MtrWel_0x26E_GearSelLostFlag)
  MtrWel_0x26E_VCU_GearSelDisp/1 -> GearDeal/5(MtrWel_0x26E_VCU_GearSelDisp)

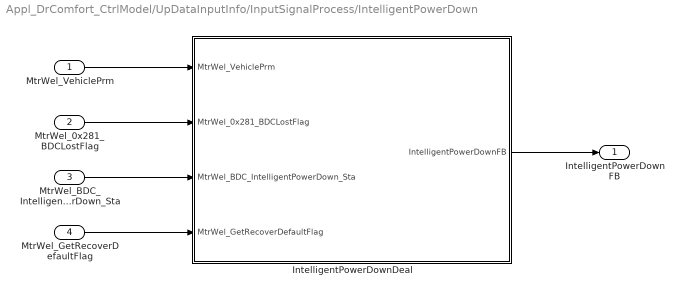
== system Appl_DrComfort_CtrlModel/UpDataInputInfo/InputSignalProcess/IntelligentPowerDown ==
  MtrWel_VehiclePrm : Inport
  MtrWel_0x281_BDCLostFlag : Inport  Port=2
  MtrWel_BDC_IntelligentPowerDown_Sta : Inport  Port=3
  MtrWel_GetRecoverDefaultFlag : Inport  Port=4
  IntelligentPowerDownDeal : Stateflow chart  TreatAsAtomicUnit=on
  IntelligentPowerDownFB : Outport
  wires:
  MtrWel_0x281_BDCLostFlag/1 -> IntelligentPowerDownDeal/2(MtrWel_0x281_BDCLostFlag)
  MtrWel_BDC_IntelligentPowerDown_Sta/1 -> IntelligentPowerDownDeal/3(MtrWel_BDC_IntelligentPowerDown_Sta)
  IntelligentPowerDownDeal/1(IntelligentPowerDownFB) -> IntelligentPowerDownFB/1
  MtrWel_VehiclePrm/1 -> IntelligentPowerDownDeal/1(MtrWel_VehiclePrm)
  MtrWel_GetRecoverDefaultFlag/1 -> IntelligentPowerDownDeal/4(MtrWel_GetRecoverDefaultFlag)

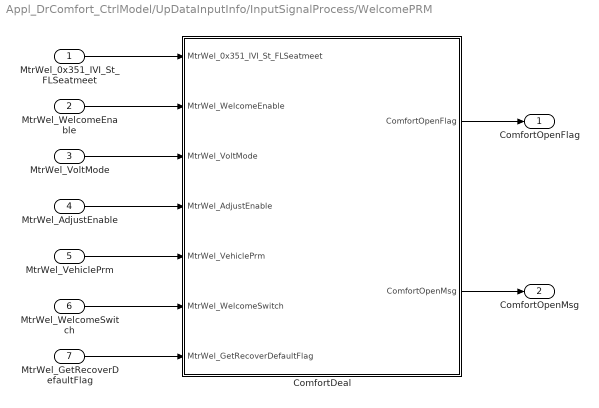
== system Appl_DrComfort_CtrlModel/UpDataInputInfo/InputSignalProcess/WelcomePRM ==
  MtrWel_0x351_IVI_St_FLSeatmeet : Inport
  MtrWel_WelcomeEnable : Inport  Port=2
  MtrWel_VoltMode : Inport  Port=3
  MtrWel_AdjustEnable : Inport  Port=4
  MtrWel_VehiclePrm : Inport  Port=5
  MtrWel_WelcomeSwitch : Inport  Port=6
  MtrWel_GetRecoverDefaultFlag : Inport  Port=7
  ComfortDeal : Stateflow chart  TreatAsAtomicUnit=on
  ComfortOpenFlag : Outport
  ComfortOpenMsg : Outport  Port=2
  wires:
  MtrWel_VoltMode/1 -> ComfortDeal/3(MtrWel_VoltMode)
  MtrWel_0x351_IVI_St_FLSeatmeet/1 -> ComfortDeal/1(MtrWel_0x351_IVI_St_FLSeatmeet)
  MtrWel_WelcomeEnable/1 -> ComfortDeal/2(MtrWel_WelcomeEnable)
  ComfortDeal/1(ComfortOpenFlag) -> ComfortOpenFlag/1
  MtrWel_AdjustEnable/1 -> ComfortDeal/4(MtrWel_AdjustEnable)
  MtrWel_VehiclePrm/1 -> ComfortDeal/5(MtrWel_VehiclePrm)
  MtrWel_WelcomeSwitch/1 -> ComfortDeal/6(MtrWel_WelcomeSwitch)
  MtrWel_GetRecoverDefaultFlag/1 -> ComfortDeal/7(MtrWel_GetRecoverDefaultFlag)
  ComfortDeal/2(ComfortOpenMsg) -> ComfortOpenMsg/1

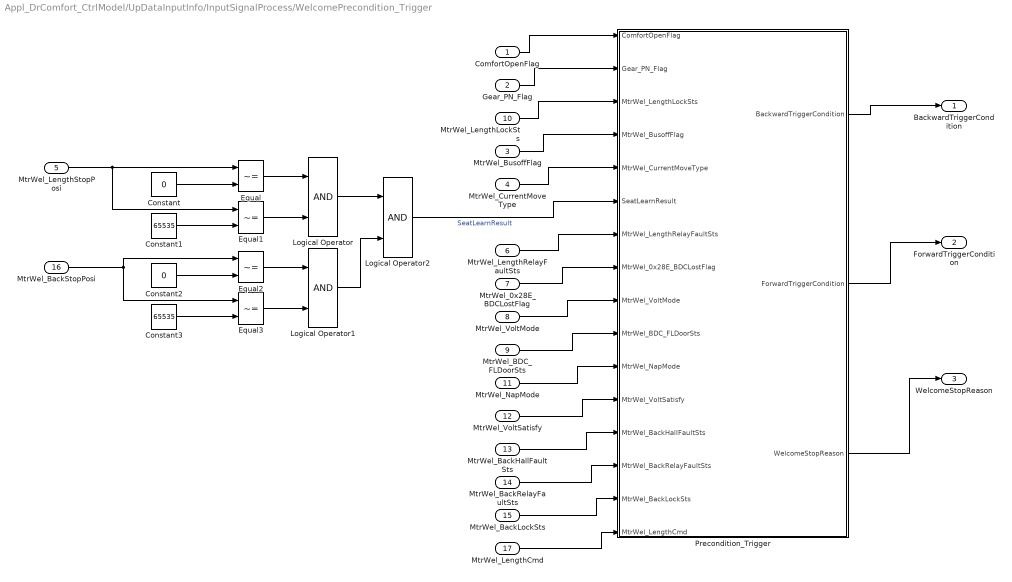
== system Appl_DrComfort_CtrlModel/UpDataInputInfo/InputSignalProcess/WelcomePrecondition_Trigger ==
  ComfortOpenFlag : Inport
  Gear_PN_Flag : Inport  Port=2
  MtrWel_BusoffFlag : Inport  Port=3
  MtrWel_CurrentMoveType : Inport  Port=4
  MtrWel_LengthStopPosi : Inport  Port=5
  MtrWel_LengthRelayFaultSts : Inport  Port=6
  MtrWel_0x28E_BDCLostFlag : Inport  Port=7
  MtrWel_VoltMode : Inport  Port=8
  MtrWel_BDC_FLDoorSts : Inport  Port=9
  MtrWel_LengthLockSts : Inport  Port=10
  MtrWel_NapMode : Inport  Port=11
  MtrWel_VoltSatisfy : Inport  Port=12
  MtrWel_BackHallFaultSts : Inport  Port=13
  MtrWel_BackRelayFaultSts : Inport  Port=14
  MtrWel_BackLockSts : Inport  Port=15
  MtrWel_BackStopPosi : Inport  Port=16
  MtrWel_LengthCmd : Inport  Port=17
  Constant : Constant  Value=0
  Constant1 : Constant  Value=65535
  Constant2 : Constant  Value=0
  Constant3 : Constant  Value=65535
  Equal{,1..3} (4 alike) : RelationalOperator  Operator=~=  OutDataTypeStr=boolean  RndMeth=Simplest
  Logical Operator : Logic  AllPortsSameDT=off  OutDataTypeStr=boolean
  Logical Operator1 : Logic  AllPortsSameDT=off  OutDataTypeStr=boolean
  Logical Operator2 : Logic  AllPortsSameDT=off  OutDataTypeStr=boolean
  Precondition_Trigger : Stateflow chart  TreatAsAtomicUnit=on
  BackwardTriggerCondition : Outport
  ForwardTriggerCondition : Outport  Port=2
  WelcomeStopReason : Outport  Port=3
  wires:
  MtrWel_BusoffFlag/1 -> Precondition_Trigger/4(MtrWel_BusoffFlag)
  Precondition_Trigger/1(BackwardTriggerCondition) -> BackwardTriggerCondition/1
  ComfortOpenFlag/1 -> Precondition_Trigger/1(ComfortOpenFlag)
  Gear_PN_Flag/1 -> Precondition_Trigger/2(Gear_PN_Flag)
  Precondition_Trigger/2(ForwardTriggerCondition) -> ForwardTriggerCondition/1
  Precondition_Trigger/3(WelcomeStopReason) -> WelcomeStopReason/1
  MtrWel_CurrentMoveType/1 -> Precondition_Trigger/5(MtrWel_CurrentMoveType)
  MtrWel_LengthRelayFaultSts/1 -> Precondition_Trigger/7(MtrWel_LengthRelayFaultSts)
  MtrWel_0x28E_BDCLostFlag/1 -> Precondition_Trigger/8(MtrWel_0x28E_BDCLostFlag)
  MtrWel_VoltMode/1 -> Precondition_Trigger/9(MtrWel_VoltMode)
  MtrWel_BDC_FLDoorSts/1 -> Precondition_Trigger/10(MtrWel_BDC_FLDoorSts)
  MtrWel_LengthLockSts/1 -> Precondition_Trigger/3(MtrWel_LengthLockSts)
  Constant1/1 -> Equal1/2
  Constant/1 -> Equal/2
  MtrWel_LengthStopPosi/1 -> Equal1/1, Equal/1
  Equal/1 -> Logical Operator/1
  Equal1/1 -> Logical Operator/2
  Logical Operator2/1 -> Precondition_Trigger/6(SeatLearnResult)  "SeatLearnResult"
  MtrWel_NapMode/1 -> Precondition_Trigger/11(MtrWel_NapMode)
  MtrWel_VoltSatisfy/1 -> Precondition_Trigger/12(MtrWel_VoltSatisfy)
  MtrWel_BackHallFaultSts/1 -> Precondition_Trigger/13(MtrWel_BackHallFaultSts)
  MtrWel_BackRelayFaultSts/1 -> Precondition_Trigger/14(MtrWel_BackRelayFaultSts)
  MtrWel_BackLockSts/1 -> Precondition_Trigger/15(MtrWel_BackLockSts)
  Logical Operator1/1 -> Logical Operator2/2
  Equal3/1 -> Logical Operator1/2
  Equal2/1 -> Logical Operator1/1
  MtrWel_BackStopPosi/1 -> Equal3/1, Equal2/1
  Constant2/1 -> Equal2/2
  Constant3/1 -> Equal3/2
  Logical Operator/1 -> Logical Operator2/1
  MtrWel_LengthCmd/1 -> Precondition_Trigger/16(MtrWel_LengthCmd)

== system Appl_DrComfort_CtrlModel/UpDataInputInfo/InputSignalProcess/WelcomePRM/ComfortDeal/SetComfortPrm ==
  in : Inport
  f : TriggerPort  TriggerType=function-call  VariantControl=(inherit)
      settings: CopyFcn=Stateflow.SLINSF.SimulinkMan.removeBlockPreDeleteFcn  PreDeleteFcn=Stateflow.SLINSF.SimulinkMan.unsafePredeleteFcn
  setAPI_type : DareLib/Dare/setAPI_type  g_funcname=Srvl_SetMemIndexDataU8  g_param=EN_MemIndex_WelcomeSwitch  g_type=uint8  g_size=-1
      settings: AttributesFormatString=%<g_funcname>  SourceProductName=Dare Library
  wires:
  in/1 -> setAPI_type/1

== system Appl_DrComfort_CtrlModel/UpDataInputInfo/InputSignalProcess/WelcomePrecondition_Trigger/Precondition_Trigger/Get_DoorSts ==
  f : TriggerPort  TriggerType=function-call  VariantControl=(inherit)
      settings: CopyFcn=Stateflow.SLINSF.SimulinkMan.removeBlockPreDeleteFcn  PreDeleteFcn=Stateflow.SLINSF.SimulinkMan.unsafePredeleteFcn
  MtrWel_WelcomeSwitch : DareLib/Dare/getAPI_type  g_funcname=Srvl_GetMemIndexDataU8  g_param=EN_MemIndex_DrDoorSts  g_type=uint8  g_size=-1
      settings: AttributesFormatString=%<g_funcname>  SourceProductName=Dare Library
  Out1 : Outport
  wires:
  MtrWel_WelcomeSwitch/1 -> Out1/1

== system Appl_DrComfort_CtrlModel/UpDataInputInfo/InputSignalProcess/WelcomePrecondition_Trigger/Precondition_Trigger/Set_DoorSts ==
  In1 : Inport
  f : TriggerPort  TriggerType=function-call  VariantControl=(inherit)
      settings: CopyFcn=Stateflow.SLINSF.SimulinkMan.removeBlockPreDeleteFcn  PreDeleteFcn=Stateflow.SLINSF.SimulinkMan.unsafePredeleteFcn
  setAPI_type : DareLib/Dare/setAPI_type  g_funcname=Srvl_SetMemIndexDataU8  g_param=EN_MemIndex_DrDoorSts  g_type=uint16  g_size=-1
      settings: AttributesFormatString=%<g_funcname>  SourceProductName=Dare Library
  wires:
  In1/1 -> setAPI_type/1

== system Appl_DrComfort_CtrlModel/UpDataInputInfo/InputSignalProcess/WelcomePrecondition_Trigger/Precondition_Trigger/Set_WelcomeUpdatePosiFlag ==
  In1 : Inport
  f : TriggerPort  TriggerType=function-call  VariantControl=(inherit)
      settings: CopyFcn=Stateflow.SLINSF.SimulinkMan.removeBlockPreDeleteFcn  PreDeleteFcn=Stateflow.SLINSF.SimulinkMan.unsafePredeleteFcn
  setAPI_type : DareLib/Dare/setAPI_type  g_funcname=Srvl_SetMemIndexDataU8  g_param=EN_MemIndex_WelcomeDrUpate  g_type=uint16  g_size=-1
      settings: AttributesFormatString=%<g_funcname>  SourceProductName=Dare Library
  wires:
  In1/1 -> setAPI_type/1

== stateflow chart Appl_DrComfort_CtrlModel/UpDataInputInfo/InputSignalProcess/IntelligentPowerDown/IntelligentPowerDownDeal ==
  state IntelligentPD_Active
    en:
    IntelligentPowerDownFB = D_Active;
  state IntelligentPD_Inactive
    en:
    IntelligentPowerDownFB = D_Inactive;
  note: /*BDC智能下电功能设置
      | 0x0:inactive
      | 0x1:active*/
  (default) -> IntelligentPD_Inactive
  IntelligentPD_Inactive -> IntelligentPD_Active : /*激活-打开*/
      | [D_Active == MtrWel_BDC_IntelligentPowerDown_Sta ...
      | && enVehTypePrm.enP20 == MtrWel_VehiclePrm]
  IntelligentPD_Active -> IntelligentPD_Inactive [order 1] : /*报文掉线 || 非激活-关闭 || 非P20车型*/
      | [TRUE == MtrWel_0x281_BDCLostFlag ...
      | || D_Inactive == MtrWel_BDC_IntelligentPowerDown_Sta ...
      | || enVehTypePrm.enP20 != MtrWel_VehiclePrm]
  IntelligentPD_Active -> IntelligentPD_Inactive [order 2] : [TRUE == MtrWel_GetRecoverDefaultFlag]
  data: MtrWel_VehiclePrm input; MtrWel_0x281_BDCLostFlag input; MtrWel_BDC_IntelligentPowerDown_Sta input; IntelligentPowerDownFB output uint8; TRUE parameter; D_Active parameter; D_Inactive parameter; MtrWel_GetRecoverDefaultFlag input

== stateflow chart Appl_DrComfort_CtrlModel/UpDataInputInfo/InputSignalProcess/BackHallChek /Chart ==
  state Check [parallel]
    en:
    BackMoreThanHall = MtrWel_BackStopPosi + (MtrWel_BackMotorSize / 4);
    du:
    BackMoreThanHall = MtrWel_BackStopPosi + (MtrWel_BackMotorSize / 4);
    settings: executionOrder=1
  state More [parallel]
    settings: executionOrder=2
    state Init
      en:
      BackMoreThanFlg = FALSE;
    state MoreThan
      en:
      BackMoreThanFlg = TRUE;
    (default) -> Init
    Init -> MoreThan : /* 大于距前止点60°位置 */
        | [MtrWel_BackHallPosi > BackMoreThanHall]
    MoreThan -> Init : /* 小于等于距前止点60°位置 */
        | [MtrWel_BackHallPosi <= BackMoreThanHall]
  data: MtrWel_BackStopPosi input; MtrWel_BackHallPosi input; MtrWel_BackMotorSize input; BackMoreThanFlg output uint8; TRUE parameter; FALSE parameter; BackMoreThanHall output uint16

== stateflow chart Appl_DrComfort_CtrlModel/LogicCtrl/LocalAdjustCtrl/WelcomeLogic ==
  state WelcomeInactive
    en:
    /*更新停止原因、清空舒适请求、纵向坐标、更新迎宾状态*/
    /*迎宾未激活：1.舒适请求 = 无； 2.迎宾坐标 = 0；*/
    WelcomeReqCMD = FALSE;
    WelcomeReqPosi = 0;
    WelcomeBackReqPosi = 0;
    WelcomeFromeInitFlag = FALSE;
    WelcomeStatus = enWelcomeSts.EN_NULL;
    Set_WelcomeStatus(WelcomeStatus);
    WelcomeRunStatus = 10;
    WelcomeInactive -> (junction 104) [order 1]
    (default) -> (junction 104)
    (junction 104) -> (junction 107) [order 1] : /*如果输入禁能原因非空，则更新输出停止原因*/
        | [enWelStopCause.EN_WelStop_NULL != WelcomeStopReason]
    (junction 104) -> (junction 109) [order 2]
    (junction 107) -> (junction 111) : {WelcomeStopReasonOut = WelcomeStopReason;
        | WelcomeRunStatus = 12;
        | /*mantis：7341存在EEPORM存储失败*/
        | Set_WelcomeStatus(WelcomeStatus);}
    (junction 111) -> (junction 109)
    (junction 109) -> (junction 114)
  state Set_WelcomeUpdatePosiFlag(In1) [function]
  state Set_WelcomeStatus(In1) [function]
  state Init
    en:
    InitTimer = 0;
    du:
    InitTimer++;
    ex:
    InitTimer = 0;
  state Set_WelcomeBWTargertPosi(In1) [function]
  state Set_WelcomeFWTargertPosi(In1) [function]
  state WelcomeActive
    state WelcomeDefault
      en:
      /*迎宾默认状态：1.舒适请求 = 无； 2.迎宾坐标 = 0；*/
      WelcomeReqCMD = FALSE;
      WelcomeReqPosi = 0;
      WelcomeBackReqPosi = 0;
    state WelcomeBackward
      state BackCheck
        (default) -> (junction 215)
        BackCheck -> (junction 215) [order 1]
        (junction 215) -> (junction 218) [order 1] : /* 靠背不满足角度需求 */
            | [BackMoreThanFlg == FALSE]
        (junction 215) -> (junction 222) [order 2]
        (junction 218) -> (junction 220) : {WelcomeBackReqPosi = BackMoreThanHall;
            | WelcomeReqCMD = TRUE;}
        (junction 220) -> (junction 222)
        (junction 222) -> (junction 225) : {WelcomeRunStatus = 14;}
      state BackwardSuccess
        en:
        /*迎宾默认状态：1.舒适请求 = 无；
        2.迎宾坐标 = 0；*/
        WelcomeReqCMD = FALSE;
        WelcomeReqPosi = 0;
        WelcomeBackReqPosi = 0;
        WelcomeRunStatus = ...
        enWelcomeRunSts.EN_Wel_BWMoveSuccess;
      state BackwardRunning
        en:
        WelcomeBackReqPosi = 0;
        WelcomeStatus = enWelcomeSts.EN_Wel_BWOngoing;
        WelcomeRunStatus = enWelcomeRunSts.EN_Wel_BWOngoing
        WelcomeReqCMD = TRUE;
        WelcomeReqPosi = LocalLengthReqPosi;
        du:
        WelcomeReqPosi = LocalLengthReqPosi;
      (default) -> BackCheck
      WelcomeBackward -> (junction 130) [order 1]
      (junction 130) -> (junction 131) [order 1] : /*有默认状态进入&&EEPROM要求更新迎宾坐标 或者数据异常 */
          | [TRUE == WelcomeFromeInitFlag ...
          | && (TRUE == MtrWel_UpdatePosiFlag ...
          | || MtrWel_LengthBWTargetPosi == 0 || MtrWel_LengthBWTargetPosi == 0xFFFF ...
          | || MtrWel_LengthFWTargetPosi == 0 || MtrWel_LengthFWTargetPosi == 0xFFFF ...
          | || MtrWel_LengthFWTargetPosi < MtrWel_LengthBWTargetPosi)]
      (junction 130) -> (junction 134) [order 2] : {LocalLengthReqPosi = MtrWel_LengthBWTargetPosi;}
      (junction 131) -> (junction 132) : {/*清初始化跳转标志位、清更新迎宾坐标标志位、更新前移坐标*/
          | WelcomeFromeInitFlag = FALSE;
          | TempPosi = MtrWel_LengthHallPosi - D_WelcomeDistance;
          | Set_WelcomeUpdatePosiFlag(FALSE);
          | Set_WelcomeFWTargertPosi(MtrWel_LengthHallPosi);}
      BackCheck -> BackwardRunning [order 1] : /* 靠背满足角度需求 */
          | [BackMoreThanFlg == TRUE]
      (junction 132) -> (junction 133) [order 1] : /*后移目标位置是否超过软止点*/
          | [TempPosi > (MtrWel_LengthStopPosi + D_SoftDistanceDrLegnth)]
      (junction 132) -> (junction 135) [order 2] : {LocalLengthReqPosi = MtrWel_LengthStopPosi + D_SoftDistanceDrLegnth;}
      (junction 133) -> (junction 136) : {LocalLengthReqPosi = TempPosi;}
      BackwardRunning -> BackwardSuccess : /*运行到后移目标位置*/
          | [enSeatAutoRunSts.EN_SEAT_SUCCESS == MtrWel_LengthAutoRunFlag]
          | /WelcomeStatus = enWelcomeSts.EN_BackwardStsSuccess;
          | WelcomeRunStatus = enWelcomeRunSts.EN_Wel_BWMoveSuccess;
          | Set_WelcomeStatus(WelcomeStatus);
      (junction 136) -> (junction 135)
      (junction 135) -> (junction 230) : {/*存储后移目标坐标*/
          | Set_WelcomeBWTargertPosi(LocalLengthReqPosi);}
      (junction 230) -> (junction 134)
      (junction 134) -> (junction 137)
    state WelcomeForward
      en:
      /*迎宾状态 = 前移*/
      /*防止突然掉电后下次不能在执行后移*/
      WelcomeStatus = enWelcomeSts.EN_Wel_FWOngoing;
      Set_WelcomeStatus(WelcomeStatus);
      /*迎宾前移：
      1.运行状态 = 前移运行中；
      2.舒适请求 = 前移；
      3.迎宾坐标 = 前移目标坐标；*/
      WelcomeRunStatus = enWelcomeRunSts.EN_Wel_FWOngoing;
      WelcomeReqCMD = TRUE;
      WelcomeReqPosi = MtrWel_LengthFWTargetPosi;
      WelcomeBackReqPosi = 0;
    (default) -> WelcomeDefault
    WelcomeDefault -> WelcomeBackward [order 1] : /*满足后移条件&&上一次未成功执行后移*/
        | [hasChangedTo(BackwardTriggerCondition,TRUE) ...
        | && enWelcomeSts.EN_BackwardStsSuccess != WelcomeStatus]
        | /WelcomeFromeInitFlag = TRUE;
    WelcomeDefault -> BackwardSuccess [order 2] : /*后移成功&&没有打断过（增加原因mantis：7341）*/
        | [enWelcomeSts.EN_BackwardStsSuccess == WelcomeStatus ...
        | && MtrWel_UpdatePosiFlag == FALSE]
    WelcomeForward -> WelcomeDefault [order 2] : /*运动到目标坐标*/
        | [enSeatAutoRunSts.EN_SEAT_SUCCESS == MtrWel_LengthAutoRunFlag]
        | /WelcomeRunStatus = enWelcomeRunSts.EN_Wel_FWMoveSuccess;
        | WelcomeStatus = enWelcomeSts.EN_ForwardStsSuccess;
        | Set_WelcomeStatus(WelcomeStatus);
    WelcomeBackward -> WelcomeForward [order 1] : /*满足前移条件*/
        | [hasChangedTo(ForwardTriggerCondition,TRUE)]
        | //WelcomeStatus = enWelcomeSts.EN_BackMovingExForWard
    WelcomeForward -> WelcomeBackward [order 1] : /*满足后移条件*/
        | [hasChangedTo(BackwardTriggerCondition,TRUE)]
        | //WelcomeStatus = enWelcomeSts.EN_ForWardMovingExBack
  (default) -> Init
  WelcomeInactive -> WelcomeActive [order 1] : /*迎宾前置条件满足*/
      | [enWelStopCause.EN_WelStop_NULL == WelcomeStopReason]
      | /WelcomeRunStatus = 11;
  WelcomeActive -> WelcomeInactive [order 1] : /*前移过程中||后移过程中前置条件不满足，下次需要更新目标坐标*/
      | [(WelcomeStatus == enWelcomeSts.EN_Wel_FWOngoing ...
      | || WelcomeStatus == enWelcomeSts.EN_Wel_BWOngoing) ...
      | && enWelStopCause.EN_WelStop_NULL != WelcomeStopReason]
      | /WelcomeStopReasonOut = WelcomeStopReason;
      | Set_WelcomeUpdatePosiFlag(TRUE);
  WelcomeActive -> WelcomeInactive [order 2] : /*存在纵向霍尔故障*/
      | [TRUE == MtrWel_LengthHallFaultSts]
      | /WelcomeStopReasonOut = enWelStopCause.EN_WelStop_HallFault;
      | Set_WelcomeUpdatePosiFlag(TRUE);
  WelcomeActive -> WelcomeInactive [order 3] : /* 靠背霍尔故障 */
      | [TRUE == MtrWel_BackHallFaultSts]
      | /WelcomeStopReasonOut = enWelStopCause.EN_WelStop_HallFault;
  WelcomeActive -> WelcomeInactive [order 4] : /*前置条件不满足，且不需要更新目标坐标*/
      | [enWelStopCause.EN_WelStop_NULL != WelcomeStopReason]
      | /WelcomeStopReasonOut = WelcomeStopReason;
  Init -> WelcomeActive : /*初始化完成，获取迎宾状态*/
      | [InitTimer > D_InitDelayTime]
      | /WelcomeStatus = MtrWel_WelcomeStatus;
      | WelcomeRunStatus = 13;
  data: In1 function_input; In1 function_input; In1 function_input; In1 function_input; BackwardTriggerCondition input; ForwardTriggerCondition input; WelcomeStopReason input; MtrWel_LengthHallFaultSts input; MtrWel_LengthStopPosi input; MtrWel_LengthHallPosi input; MtrWel_LengthFWTargetPosi input; MtrWel_LengthBWTargetPosi input; MtrWel_LengthAutoRunFlag input; TRUE parameter; FALSE parameter; MtrWel_WelcomeStatus input; D_WelcomeDistance parameter; D_SoftDistanceDrLegnth parameter; TempPosi local uint16; WelcomeFromeInitFlag local uint8; WelcomeStopReasonOut output uint8; WelcomeStatus local Enum: enWelcomeSts; WelcomeRunStatus output uint8; WelcomeReqCMD output uint8; WelcomeReqPosi output uint16; InitTimer local uint8; MtrWel_UpdatePosiFlag input; MtrWel_BackHallFaultSts input; D_InitDelayTime parameter; BackMoreThanFlg input; BackMoreThanHall input; WelcomeBackReqPosi output uint16; LocalLengthReqPosi local uint16

== stateflow chart Appl_DrComfort_CtrlModel/UpDataInputInfo/InputSignalProcess/GearMessageDeal/GearDeal ==
  state Gear_Not_PN
    en:
    Gear_PN_Flag = FALSE;
    note: /*Gear selector position
        | 档位状态
        | 0x0:P
        | 0x1:Reserved
        | 0x2:Reserved
        | 0x3:Reserved
        | 0x4:Reserved
        | 0x5:D
        | 0x6:N
        | 0x7:R
        | 0xF:Fault Value*/
  state Gear_PN
    en:
    Gear_PN_Flag = TRUE;
  (default) -> Gear_Not_PN
  Gear_Not_PN -> Gear_PN [order 1] : /*油车报文掉线 || PN档报文*/
      | [(TRUE == MtrWel_0x238_GearLostFlag ...
      | || 0 == MtrWel_0x238_TCU_GearSelDisp ...
      | || 6 == MtrWel_0x238_TCU_GearSelDisp) ...
      | && FALSE == MtrWel_P20_PHEV_EngineCfg]
  Gear_PN -> Gear_Not_PN [order 1] : /*油车报文在线 && 非PN档报文*/
      | [(5 == MtrWel_0x238_TCU_GearSelDisp ...
      | || 7 == MtrWel_0x238_TCU_GearSelDisp ...
      | || 0xF == MtrWel_0x238_TCU_GearSelDisp) ...
      | && FALSE == MtrWel_P20_PHEV_EngineCfg]
  Gear_Not_PN -> Gear_PN [order 2] : /*电车报文掉线 || PN档报文*/
      | [(TRUE == MtrWel_0x26E_GearSelLostFlag ...
      | || 0 == MtrWel_0x26E_VCU_GearSelDisp ...
      | || 6 == MtrWel_0x26E_VCU_GearSelDisp) ...
      | && FALSE != MtrWel_P20_PHEV_EngineCfg]
  Gear_PN -> Gear_Not_PN [order 2] : /*电车报文掉线 || 非PN档报文*/
      | [(5 == MtrWel_0x26E_VCU_GearSelDisp ...
      | || 7 == MtrWel_0x26E_VCU_GearSelDisp ...
      | || 0xF == MtrWel_0x26E_VCU_GearSelDisp) ...
      | && FALSE != MtrWel_P20_PHEV_EngineCfg]
  data: MtrWel_0x238_GearLostFlag input; MtrWel_0x238_TCU_GearSelDisp input; Gear_PN_Flag output uint8; TRUE parameter; FALSE parameter; MtrWel_P20_PHEV_EngineCfg input; MtrWel_0x26E_GearSelLostFlag input; MtrWel_0x26E_VCU_GearSelDisp input
